simulink model "Model4"  (R2020a)
settings: Solver=VariableStepAuto  StartTime=0.0  StopTime=1  RelTol=1e-3
model workspace (MAT data in the model file):
  pathDelays = [0 2e-07 4e-07 8e-07]
undefined symbols (not defined in the file or in its folder): doppler, Pavg, pskmod
libraries: commutil2 x4, commdigbbndpm3 x3, commchan3 x2, commsink2 x2, commrandsrc3 x1
settings Model: Creator=esha_  LastModifiedBy=esha_

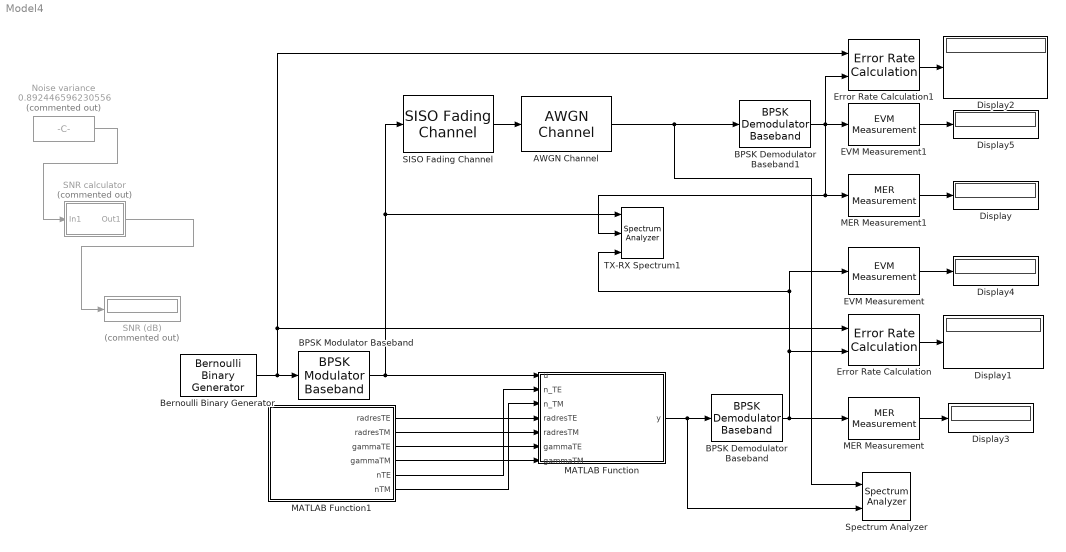
== system Model4 ==
  AWGN Channel : commchan3/AWGN Channel  InputProcessing=Columns as channels (frame based)  seed=67  noiseMode="Signal to noise ratio  (SNR)"  EbNodB=1  EsNodB=10  SNRdB=0  bitsPerSym=1  Ps=0.001  Tsym=0.000000065  variance=1
  BPSK Demodulator Baseband : commdigbbndpm3/BPSK Demodulator Baseband  DecType=Hard decision  VarSource=Dialog  Variance=1  Ph=0  outDtype=Inherit via internal rule  derotateFactorWordLen=16  derotateFactorDataTypeStr=Inherit: Same word length as input  derotateFactorLastDataTypeStr=Inherit: Same word length as input
  BPSK Demodulator Baseband1 : commdigbbndpm3/BPSK Demodulator Baseband  DecType=Hard decision  VarSource=Dialog  Variance=1  Ph=0  outDtype=Inherit via internal rule  derotateFactorWordLen=16  derotateFactorDataTypeStr=Inherit: Same word length as input  derotateFactorLastDataTypeStr=Inherit: Same word length as input
  BPSK Modulator Baseband : commdigbbndpm3/BPSK Modulator Baseband  Ph=0  outDtype=double  outWordLen=16  outUDDataType=sfix(16)  outFracLenMode=Best precision  outFracLen=15  outDataTypeStr=double  outLastDataTypeStr=double
  Bernoulli Binary Generator : commrandsrc3/Bernoulli Binary Generator  ProbabilityOfZero=0.5  SeedSource=Parameter  Seed=61  SampleTime=1.302083333333333e-07  SamplesPerFrame=1E4  OutputDataType=double  SimulateUsing=Code generation
  Display{,1..5} (6 alike) : Display
  EVM Measurement : commutil2/EVM Measurement  Normalization=Average reference signal power  AverageConstellationPower=1  PeakConstellationPower=1  ReferenceSignalSource=Estimated from reference constellation  ReferenceConstellation=pskmod((0:1),2,0)  MeasurementIntervalSource=Input length  MeasurementInterval=100  AveragingDimensions=1  MaximumEVMOutputPort=off  XPercentileEVMOutputPort=off  XPercentileValue=95  SymbolCountOutputPort=on  SimulateUsing=Interpreted execution
      settings: SourceProductBaseCode=CM
  EVM Measurement1 : commutil2/EVM Measurement  Normalization=Average reference signal power  AverageConstellationPower=1  PeakConstellationPower=1  ReferenceSignalSource=Estimated from reference constellation  ReferenceConstellation=pskmod((0:1),2,0)  MeasurementIntervalSource=Input length  MeasurementInterval=100  AveragingDimensions=1  MaximumEVMOutputPort=off  XPercentileEVMOutputPort=off  XPercentileValue=95  SymbolCountOutputPort=on  SimulateUsing=Interpreted execution
      settings: SourceProductBaseCode=CM
  Error Rate Calculation : commsink2/Error Rate Calculation  N=0  st_delay=0  cp_mode=Entire frame  subframe=[]  PMode=Port  WsName=ErrorVec  RsMode2=off  stop=off  numErr=100  maxBits=1e6
  Error Rate Calculation1 : commsink2/Error Rate Calculation  N=0  st_delay=0  cp_mode=Entire frame  subframe=[]  PMode=Port  WsName=ErrorVec  RsMode2=off  stop=off  numErr=100  maxBits=1e6
  MATLAB Function : MATLAB Function  TreatAsAtomicUnit=on
  MATLAB Function1 : MATLAB Function  TreatAsAtomicUnit=on
  MER Measurement : commutil2/MER Measurement  ReferenceSignalSource=Estimated from reference constellation  ReferenceConstellation=pskmod((0:1),2,0)  MeasurementIntervalSource=Input length  MeasurementInterval=100  AveragingDimensions=1  MinimumMEROutputPort=off  XPercentileMEROutputPort=off  XPercentileValue=95  SymbolCountOutputPort=off  SimulateUsing=Interpreted execution
      settings: SourceProductBaseCode=CM
  MER Measurement1 : commutil2/MER Measurement  ReferenceSignalSource=Estimated from reference constellation  ReferenceConstellation=pskmod((0:1),2,0)  MeasurementIntervalSource=Input length  MeasurementInterval=100  AveragingDimensions=1  MinimumMEROutputPort=off  XPercentileMEROutputPort=off  XPercentileValue=95  SymbolCountOutputPort=off  SimulateUsing=Interpreted execution
      settings: SourceProductBaseCode=CM
  Noise variance : Constant  Commented=on  Value=0.892446596230556  VectorParams1D=off  OutDataTypeStr=Inherit: Inherit via back propagation  SampleTime=1.302083333333333e-3
  SISO Fading Channel : commchan3/SISO Fading Channel  InheritSampleRate=on  SampleRate=1  PathDelays="[0     2E-9]"  AveragePathGains="[-60     -60]"  NormalizePathGains=on  FadingDistribution=Rayleigh  KFactor=3  DirectPathDopplerShift=0  DirectPathInitialPhase=0  MaximumDopplerShift=0  DopplerSpectrum=doppler('Jakes')  RandomStream=mt19937ar with seed  Seed=61  PathGainsOutputPort=off  ChannelFilterDelayOutputPort=off  SimulateUsing=Interpreted execution  Visualization=Frequency response  PathsForDopplerDisplay=1  SamplesToDisplay=100%
  SNR calculator : Subsystem  Commented=on
      mask Display: fprintf('SNR\nCalculator')
  SNR (dB) : Display  Commented=on
  Spectrum Analyzer : SpectrumAnalyzer  NumInputPorts=2
  TX-RX Spectrum1 : SpectrumAnalyzer  NumInputPorts=3
  wires:
  MATLAB Function1/2(radresTM) -> MATLAB Function/5(radresTM)
  MATLAB Function1/1(radresTE) -> MATLAB Function/4(radresTE)
  BPSK Modulator Baseband/1 -> MATLAB Function/1(u), SISO Fading Channel/1, TX-RX Spectrum1/1
  MATLAB Function/1(y) -> Spectrum Analyzer/2, BPSK Demodulator Baseband/1
  Error Rate Calculation/1 -> Display1/1
  Bernoulli Binary Generator/1 -> Error Rate Calculation1/1, Error Rate Calculation/1, BPSK Modulator Baseband/1
  MATLAB Function1/4(gammaTM) -> MATLAB Function/7(gammaTM)
  BPSK Demodulator Baseband/1 -> MER Measurement/1, Error Rate Calculation/2, EVM Measurement/1, TX-RX Spectrum1/3
  MATLAB Function1/3(gammaTE) -> MATLAB Function/6(gammaTE)
  Error Rate Calculation1/1 -> Display2/1
  AWGN Channel/1 -> Spectrum Analyzer/1, BPSK Demodulator Baseband1/1
  BPSK Demodulator Baseband1/1 -> EVM Measurement1/1, Error Rate Calculation1/2, MER Measurement1/1, TX-RX Spectrum1/2
  EVM Measurement1/1 -> Display5/1
  MATLAB Function1/5(nTE) -> MATLAB Function/2(n_TE)
  MATLAB Function1/6(nTM) -> MATLAB Function/3(n_TM)
  MER Measurement/1 -> Display3/1
  MER Measurement1/1 -> Display/1
  EVM Measurement/1 -> Display4/1
  SISO Fading Channel/1 -> AWGN Channel/1
  Noise variance/1 -> SNR calculator/1(In1)
  SNR calculator/1(Out1) -> SNR (dB)/1

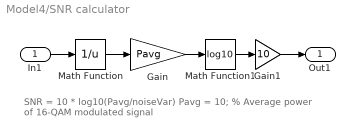
== system Model4/SNR calculator ==
  note: SNR = 10 * log10(Pavg/noiseVar)
      |
      | Pavg = 10; % Average power of 16-QAM modulated signal
  In1 : Inport
  Gain : Gain  Gain=Pavg
  Gain1 : Gain  Gain=10
  Math Function : Math  Operator=reciprocal  SignedPower=on  SaturateOnIntegerOverflow=on
  Math Function1 : Math  Operator=log10  SignedPower=on  SaturateOnIntegerOverflow=on
  Out1 : Outport
  wires:
  In1/1 -> Math Function/1
  Math Function/1 -> Gain/1
  Gain/1 -> Math Function1/1
  Math Function1/1 -> Gain1/1
  Gain1/1 -> Out1/1

== matlab function Model4/MATLAB Function1 ==
  data: radresTE output; radresTM output; gammaTE output; gammaTM output; nTE output; nTM output
function [radresTE, radresTM, gammaTE, gammaTM, nTE, nTM] = fcn()
nTE1 = load('nTE.mat');
nTE = nTE1.n_TE;
nTM1 = load('nTM.mat');
nTM = nTM1.n_TM;
radresTE1 = load('radresTE.mat');
radresTE = radresTE1.radresTES;
radresTM1 = load('radresTM.mat');
radresTM = radresTM1.radresTMS;
gammaTE1 = load('gammaTE.mat');
gammaTE = gammaTE1.gammaTES;
gammaTM1 = load('gammaTM.mat');
gammaTM = gammaTM1.gammaTMS;
end

== matlab function Model4/MATLAB Function ==
  data: y output; u input; n_TE input; n_TM input; radresTE input; radresTM input; gammaTE input; gammaTM input
function y = fcn(u,n_TE, n_TM, radresTE, radresTM, gammaTE, gammaTM)
freq = 59E9:4E6:60E9; 
% n_TE = 0;
% n_TM = 17;
Zo=50;
WGlen = 5;

radreacTE = imag(hilbert(radresTE));
radreacTM = imag(hilbert(radresTM));
antresTE = zeros(1,length(freq));
antresTM = zeros(1,length(freq));
antreacTE = zeros(1,length(freq));
antreacTM = zeros(1,length(freq));
antimpTE = zeros(1,length(freq)) + 1i*zeros(1,length(freq));
antimpTM = zeros(1,length(freq)) + 1i*zeros(1,length(freq));
TEmodeimp = zeros(length(freq), length(n_TE)) + 1i*zeros(length(freq), length(n_TE));
TMmodeimp = zeros(length(freq), length(n_TM)) + 1i*zeros(length(freq), length(n_TM));
channel = zeros(1,length(freq)) + 1i*zeros(1,length(freq));
for fi=1:length(freq)
    antresTE(fi) = sum(radresTE(fi,:));
    antresTM(fi) = sum(radresTM(fi,:));
    antreacTE(fi) = sum(radreacTE(fi,:));
    antreacTM(fi) = sum(radreacTM(fi,:));
    antimpTE(fi) = antresTE(fi) +1i*antreacTE(fi);
    antimpTM(fi) = antresTM(fi) +1i*antreacTM(fi);
    for n = 1:length(n_TE)
        TEmodeimp(fi,n)=radresTE(fi,n)+1i*radreacTE(fi,n);
    end
    for n = 1:length(n_TM)
        TMmodeimp(fi,n)=radresTM(fi,n)+1i*radreacTM(fi,n);
    end    
end
for fi=1:length(freq)
    TsTE = diag(exp(-1*gammaTE(fi,:)*WGlen));
    chTEmode = TEmodeimp(fi,:)*TsTE;
    TsTM = diag(exp(-1*gammaTM(fi,:)*WGlen));
    chTMmode = TMmodeimp(fi,:)*TsTM;
%     channel(fi) = ((2*Zo)/(abs(Zo + antimpTM(fi))^2))*...
%         (sum(chTMmode));
    channel(fi) = ((2*Zo)/(abs(antimpTM(fi) + Zo + antimpTE(fi))^2))*...
        (sum(chTEmode)+sum(chTMmode));
end
%uu = u';
 cchanel = ((abs(channel)).^2);
 y = zeros(length(u),1);
 for ui = 1:length(u)
     y(ui) = sum(u(ui)*cchanel);
 end
%y = uu.*(cchanel);
% y = conv(u,(abs(channel)).^2,'same');
%y = channel;
